simulink model "test_mpu6050"  (R2024b)
settings: Solver=FixedStepAuto  StartTime=0.0  StopTime=1000  FixedStep=dt  RelTol=1e-3
model workspace (MAT data in the model file):
  dt = Simulink.Parameter
  dt.Value = 0.001
  dt.Complexity = 'real'
  dt.Dimensions = [1 1]
  dt.DataType = 'auto'
libraries: simulink x2
settings Model: ExtModeTrigDuration=2  Creator=schwmaxi  LastModifiedBy=schwmaxi
settings SolverCC: PositivePriorityOrder=on
settings OptimizationCC: BlockReduction=off  BooleanDataType=off  DefaultParameterBehavior=Inlined  EnhancedBackFolding=on  PassReuseOutputArgsAs=Individual arguments  ZeroExternalMemoryAtStartup=off  ZeroInternalMemoryAtStartup=off  MaxStackSize=200000  OptimizeBlockOrder=speed  DifferentSizesBufferReuse=on  OptimizationCustomize=off  EfficientTunableParamExpr=on
settings DebuggingCC: SaveWithParameterizedLinksMsg=none  UnderspecifiedInitializationDetection=Classic  MergeDetectMultiDrivingBlocksExec=none  SignalResolutionControl=TryResolveAllWithWarning  ParameterTunabilityLossMsg=error
settings HardwareCC: ProdBitPerPointer=32  ProdBitPerSizeT=32  ProdBitPerPtrDiffT=32  ProdLargestAtomicInteger=Long  ProdLargestAtomicFloat=Double  ProdWordSize=32  ProdLongLongMode=on  ProdHWDeviceType=ARM Compatible->ARM Cortex-A (32-bit)  UseEmbeddedCoderFeatures=off
settings ModelReferenceCC: PropagateSignalLabelsOutOfModel=off
settings RTWCC: Description=Embedded Coder  SystemTargetFile=ert.tlc  HardwareBoard=Raspberry Pi  TLCOptions="-aInlineSetEventsForThisBaseRateFcn=TLC_FALSE -aSuppressMultiTaskScheduler=TLC_FALSE  -aRateBasedStepFcn=0"  TemplateMakefile=ert_default_tmf  Toolchain=GNU GCC Embedded Linux
settings CodeAppCC: ForceParamTrailComments=on  IgnoreCustomStorageClasses=off  OperatorAnnotations=on  SimulinkDataObjDesc=on  SFDataObjDesc=on  InsertBlockDesc=on
settings ERTTargetCC: SupportNonInlinedSFcns=on  SupportVariableSizeSignals=on  ExtModeTransport=2  ExtModeStaticAlloc=on  ExtModeMexFile=ext_xcp  ExtModeIntrfLevel=Level2 - Open

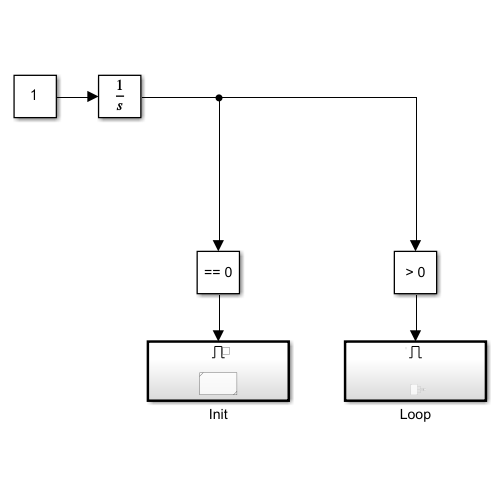
[thumbnail: Simulink's stored preview of the top-level diagram]
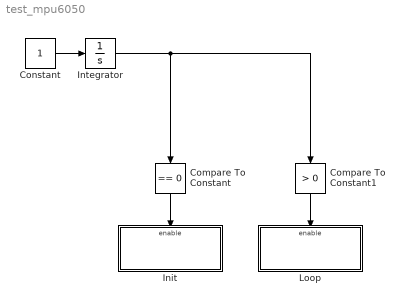
== system test_mpu6050 ==
  Compare To Constant : simulink/Logic and Bit Operations/Compare To Constant  relop===  const=0  OutDataTypeStr=boolean
  Compare To Constant1 : simulink/Logic and Bit Operations/Compare To Constant  relop=>  const=0  OutDataTypeStr=boolean
  Constant : Constant
  Init : Subsystem  TreatAsAtomicUnit=on
  Integrator : Integrator
  Loop : Subsystem  TreatAsAtomicUnit=on
  wires:
  Compare To Constant/1 -> Init/Enable
  Integrator/1 -> Compare To Constant1/1, Compare To Constant/1
  Constant/1 -> Integrator/1
  Compare To Constant1/1 -> Loop/Enable

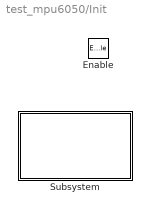
== system test_mpu6050/Init ==
  Enable : EnablePort
  Subsystem : Subsystem  ReferencedSubsystem=InitIMU

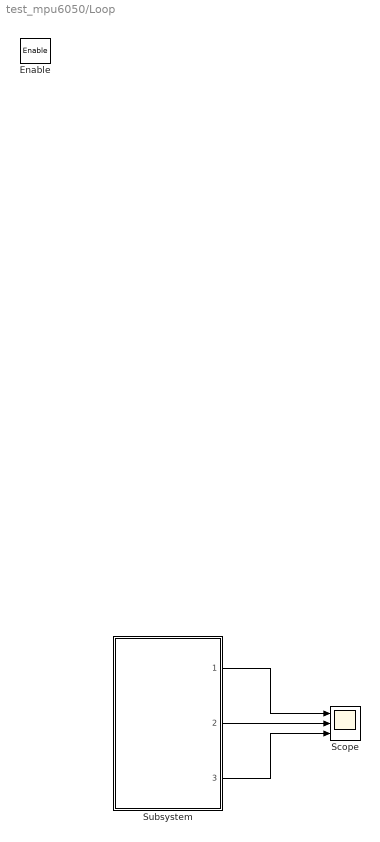
== system test_mpu6050/Loop ==
  Enable : EnablePort
  Scope : Scope  NumInputPorts=3
  Subsystem : Subsystem  ReferencedSubsystem=IMU
  wires:
  Subsystem/2 -> Scope/2
  Subsystem/1 -> Scope/1
  Subsystem/3 -> Scope/3
